simulink model "problem2"  (R2020a)
settings: Solver=VariableStepAuto  StartTime=0.0  StopTime=10.0  RelTol=1e-3
settings Model: Creator=kasutav  LastModifiedBy=kasutav

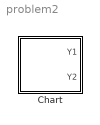
== system problem2 ==
  Chart : Stateflow chart  TreatAsAtomicUnit=on

== stateflow chart problem2/Chart ==
  state StopGo
    Y1=RED;
    Y2=GREEN;
  state StopReady
    Y1=RED;
    Y2=YELLOW;
  state ReadyStop
    Y1=YELLOW;
    Y2=RED;
  state GoStop
    Y1=GREEN;
    Y2=RED;
  (default) -> StopGo
  StopGo -> StopReady : after(20,tick)
  ReadyStop -> StopGo : after(10,tick)
  StopReady -> GoStop : after(10,tick)
  GoStop -> ReadyStop : after(20,tick)
  data: GREEN constant double =3; YELLOW constant double =2; RED constant double =1; Y1 output; Y2 output
